simulink model "ModelAgriAuto"  (R2022a)
settings: Solver=FixedStepAuto  StartTime=0.0  StopTime=6240  FixedStep=0.05  MaxStep=0.1  RelTol=1e-3
model workspace (MAT data in the model file):
  PlowHectare = 1.925
values from neighbouring files (symbols this model uses):
  C_rate = 3    [start_function.m]
  Compaction = 0    [start_function.m]
  CyclesIn = CyclesIn+CyclesOut(end)    [start_function.m]
  Degradation = 2    [start_function.m]
  FailRate = 29700000    [start_function.m]
  FieldEff = 0.8    [start_function.m]
  ForceCorrVar = 0.85    [start_function.m]
  Fuel = 3    [start_function.m]
  Mass = 10550    [start_function.m]
  n = n+1    (= 2)    [start_function.m]
  v_field = 5    [start_function.m]
  Weather_crit = 3    [start_function.m]
  WorkingHours = 10    [start_function.m]
undefined symbols (not defined in the file or in its folder): Battery, BatteryNo, Charger, ChargerNo, DField, m, Power, Soil, TractorNo, Year
libraries: simulink x2
(part 3 of 3)

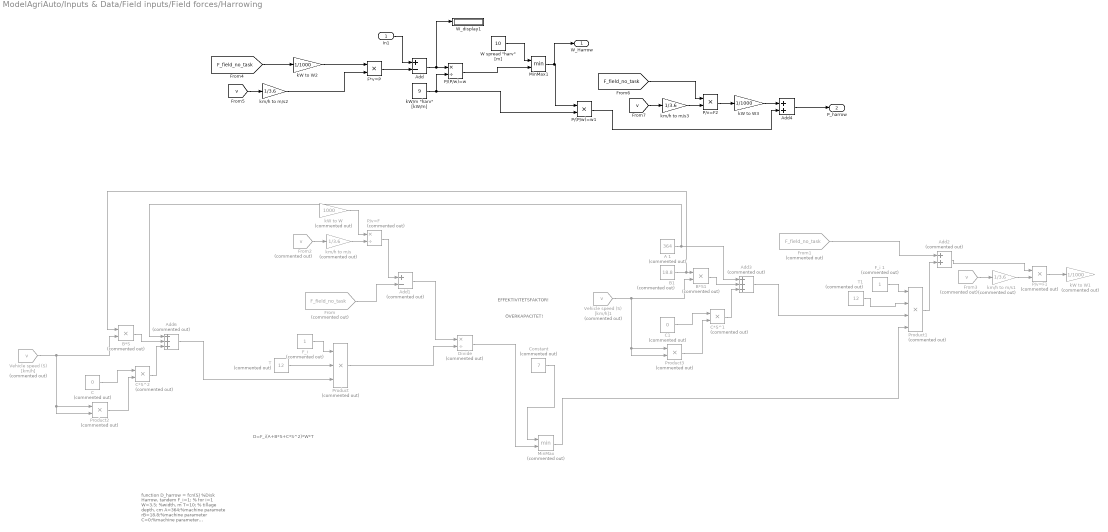
== system ModelAgriAuto/Inputs & Data/Field inputs/Field forces/Harrowing ==
  note: function D_harrow = fcn(S)
      |
      | %Disk Harrow, tandem
      | F_i=1; % for i=1
      | W=3.5; %width, m
      | T=10; % tillage depth, cm
      | A=364;%machine paramete
      | rB=18.8;%machine parameter
      | C=0;%machine parameter
      |
      | D_harrow=F_i*(A+B*S+C*S^2)*W*T;
  note: EFFEKTIVITETSFAKTOR!
  note: ÖVERKAPACITET!
  note: D=F_i(A+B*S+C*S^2)*W*T
  In1 : Inport
  A 1 : Constant  Commented=on  Value=364
  Add : Sum  Inputs=+-
  Add1 : Sum  Commented=on  Inputs=+-
  Add2 : Sum  Commented=on
  Add3 : Sum  Commented=on  Inputs=+++
  Add4 : Sum
  Add6 : Sum  Commented=on  Inputs=+++
  B*S : Product  Commented=on
  B*S1 : Product  Commented=on
  B1 : Constant  Commented=on  Value=18.8
  C : Constant  Commented=on  Value=0
  C*S^1 : Product  Commented=on
  C*S^2 : Product  Commented=on
  C1 : Constant  Commented=on  Value=0
  Constant : Constant  Commented=on  Value=7
  Divide : Product  Commented=on  Inputs=*/
  F*v=P : Product  Inputs=**
  "F_i " : Constant  Commented=on
  F_i 1 : Constant  Commented=on
  From : From  Commented=on  GotoTag=F_field_no_task  TagVisibility=global
  From1 : From  Commented=on  GotoTag=F_field_no_task  TagVisibility=global
  From2 : From  Commented=on  GotoTag=v  TagVisibility=global
  From3 : From  Commented=on  GotoTag=v  TagVisibility=global
  MinMax : MinMax  Commented=on  Inputs=2
  MinMax1 : MinMax  Inputs=2
  P/(P/w)=w : Product  Inputs=*/
  P/(P/w)=w1 : Product  Inputs=**
  P/v=F : Product  Commented=on  Inputs=*/
  P/v=F1 : Product  Commented=on  Inputs=**
  P/v=F2 : Product  Inputs=**
  Product : Product  Commented=on  Inputs=3
  Product1 : Product  Commented=on  Inputs=4
  Product2 : Product  Commented=on
  Product3 : Product  Commented=on
  T : Constant  Commented=on  Value=12
  T1 : Constant  Commented=on  Value=12
  Vehicle speed (S) [km/h] : From  Commented=on  GotoTag=v  TagVisibility=global
  Vehicle speed (S) [km/h]1 : From  Commented=on  GotoTag=v  TagVisibility=global
  "W spread \"harv\" [m]" : Constant  Value=10
  W_display1 : Display
  kW to W : Gain  Commented=on  Gain=1000
  kW to W1 : Gain  Commented=on  Gain=1/1000
  kW to W2 : Gain  Gain=1/1000
  kW to W3 : Gain  Gain=1/1000
  "kW/m \"harv\" [kW/m] " : Constant  Value=9
  km/h to m/s : Gain  Commented=on  Gain=1/3.6
  km/h to m/s1 : Gain  Commented=on  Gain=1/3.6
  km/h to m/s2 : Gain  Gain=1/3.6
  km/h to m/s3 : Gain  Gain=1/3.6
  W_Harrow : Outport  VectorParamsAs1DForOutWhenUnconnected=off
  P_harrow : Outport  Port=2  VectorParamsAs1DForOutWhenUnconnected=off
  wires:
  Product2/1 -> C*S^2/2
  T/1 -> Product/2
  C/1 -> C*S^2/1
  C*S^2/1 -> Add6/3
  From/1 -> Add1/2
  km/h to m/s/1 -> P/v=F/2
  kW to W/1 -> P/v=F/1
  Vehicle speed (S) [km/h]/1 -> Product2/2, Product2/1, B*S/2
  Add1/1 -> Divide/1
  "F_i "/1 -> Product/1
  Product/1 -> Divide/2
  Add6/1 -> Product/3
  B*S/1 -> Add6/2
  From2/1 -> km/h to m/s/1
  B1/1 -> B*S/1, B*S1/1
  A 1/1 -> Add6/1, Add3/1
  Divide/1 -> MinMax/2
  Constant/1 -> MinMax/1
  P/v=F/1 -> Add1/1
  B*S1/1 -> Add3/2
  Product3/1 -> C*S^1/2
  C*S^1/1 -> Add3/3
  F_i 1/1 -> Product1/1
  C1/1 -> C*S^1/1
  Vehicle speed (S) [km/h]1/1 -> Product3/2, Product3/1, B*S1/2
  Add2/1 -> P/v=F1/1
  T1/1 -> Product1/2
  MinMax/1 -> Product1/4
  Add3/1 -> Product1/3
  Product1/1 -> Add2/2
  From1/1 -> Add2/1
  km/h to m/s1/1 -> P/v=F1/2
  From3/1 -> km/h to m/s1/1
  P/v=F1/1 -> kW to W1/1
  F*v=P/1 -> Add/2
  "W spread \"harv\" [m]"/1 -> MinMax1/1
  [F_field_no_task] -> kW to W2/1
  [v] -> km/h to m/s2/1
  P/(P/w)=w/1 -> MinMax1/2
  km/h to m/s2/1 -> F*v=P/2
  kW to W2/1 -> F*v=P/1
  Add/1 -> W_display1/1, P/(P/w)=w/1
  P/(P/w)=w1/1 -> Add4/2
  MinMax1/1 -> W_Harrow/1, P/(P/w)=w1/1
  "kW/m \"harv\" [kW/m] "/1 -> P/(P/w)=w1/2, P/(P/w)=w/2
  [v] -> km/h to m/s3/1
  [F_field_no_task] -> P/v=F2/1
  km/h to m/s3/1 -> P/v=F2/2
  P/v=F2/1 -> kW to W3/1
  kW to W3/1 -> Add4/1
  In1/1 -> Add/1
  Add4/1 -> P_harrow/1

== system ModelAgriAuto/Inputs & Data/Field inputs/Field forces/Motion resistance  ==
  note: %rho =MR/W=1/B_n+0.04+ 0.5*s/sqrtBn
  Add : Sum  Inputs=+++
  B_n : Constant  Value=55
  Constant : Constant  Value=1000
  Constant1 : Constant
  Constant2 : Constant  Value=0.04
  Constant4 : Constant  Value=0.5
  Divide : Product  Inputs=*/
  Divide1 : Product  Inputs=**/
  Divide2 : Product  Inputs=/*
  Product1 : Product
  Product2 : Product
  Sqrt : Sqrt
  g : Constant  Value=9.81
  kN to N : Gain  Gain=1000
  "slippage " : Constant  Value=0.2
  tag scope: MR=global
  wires:
  B_n/1 -> Sqrt/1, Divide/2
  Constant1/1 -> Divide/1
  [m] -> Divide1/1
  g/1 -> Divide1/2
  Divide/1 -> Add/1
  Constant2/1 -> Add/2
  Constant4/1 -> Product1/1
  "slippage "/1 -> Product1/2
  Sqrt/1 -> Divide2/1
  Product1/1 -> Divide2/2
  Divide2/1 -> Add/3
  Add/1 -> Product2/2
  Divide1/1 -> Product2/1
  Product2/1 -> kN to N/1
  Constant/1 -> Divide1/3
  kN to N/1 -> [MR]

== system ModelAgriAuto/Inputs & Data/Field inputs/Field forces/Pest Spreading ==
  note: EMMA och Engström/Lagnelöv 2017
  In2 : Inport
  Add : Sum  Inputs=+-
  Add4 : Sum
  Constant1 : Constant  Commented=on  Value=3.1159
  Constant2 : Constant  Commented=on  Value=2.33
  F*v=P : Product  Inputs=**
  MinMax : MinMax  Inputs=2
  "P spread \"fastgödsel\" [kW]" : Constant  Commented=on  Value=48
  "P spread \"kletgödsel\" [kW]" : Constant  Commented=on  Value=43
  "P spread \"konstgödsel\" [kW]" : Constant  Commented=on  Value=16
  "P spread \"urin\" [kW] " : Constant  Commented=on  Value=28
  P/(P/w)=w : Product  Inputs=*/
  P/(P/w)=w1 : Product  Inputs=**
  P/v=F2 : Product  Inputs=**
  "W spread \"art. fert.\" [m]" : Constant  Value=24
  "W spread \"fastgödsel\" [m]" : Constant  Commented=on  Value=6
  "W spread \"kletgödsel\" [m]1" : Constant  Commented=on  Value=13.8
  "W spread \"konstgödsel\" [m]" : Constant  Commented=on  Value=22
  "W spread \"urin\" [m]" : Constant  Commented=on  Value=12
  W_display1 : Display
  "ha/h \"kletgödsel\" " : Constant  Commented=on  Value=6.9
  "ha/h \"konstgödsel\" " : Constant  Commented=on  Value=11
  kW to W1 : Gain  Gain=1/1000
  kW to W3 : Gain  Gain=1/1000
  kW/m : Constant  Commented=on  Value=0.7273
  "kW/m \"Urin\" [kW/m] " : Constant  Value=2.2917
  km/h to m/s1 : Gain  Gain=1/3.6
  km/h to m/s3 : Gain  Gain=1/3.6
  kw/m : Constant  Commented=on  Value=8
  W_spread : Outport  VectorParamsAs1DForOutWhenUnconnected=off
  P_spread : Outport  Port=2  VectorParamsAs1DForOutWhenUnconnected=off
  wires:
  In2/1 -> Add/1
  [F_field_no_task] -> kW to W1/1
  MinMax/1 -> P/(P/w)=w1/1, W_spread/1
  "W spread \"art. fert.\" [m]"/1 -> MinMax/1
  kW to W1/1 -> F*v=P/1
  [v] -> km/h to m/s1/1
  km/h to m/s1/1 -> F*v=P/2
  F*v=P/1 -> Add/2
  Add/1 -> W_display1/1, P/(P/w)=w/1
  "kW/m \"Urin\" [kW/m] "/1 -> P/(P/w)=w1/2, P/(P/w)=w/2
  P/(P/w)=w/1 -> MinMax/2
  P/v=F2/1 -> kW to W3/1
  kW to W3/1 -> Add4/1
  [F_field_no_task] -> P/v=F2/1
  km/h to m/s3/1 -> P/v=F2/2
  [v] -> km/h to m/s3/1
  P/(P/w)=w1/1 -> Add4/2
  Add4/1 -> P_spread/1

== system ModelAgriAuto/Inputs & Data/Field inputs/Field forces/Plowing ==
  note: Moldboard Plow
  note: W=1; %width, m
      | F_i=1; % for i=1
      | T=20; % tillage depth, cm
      | A=652;%machine paramete
      | B=0;%machine parameter
      | C=5.1;%machine parameter
  note: D=F_i(A+B*S+C*S^2)*W*T
  In1 : Inport
  "A " : Constant  Value=652
  Add1 : Sum  Inputs=+-
  Add2 : Sum
  Add6 : Sum  Inputs=+++
  B : Constant  Value=0
  B*S : Product
  C : Constant  Value=5.1
  C*S^2 : Product
  Constant : Constant  Value=6
  Display : Display
  Divide : Product  Inputs=*/
  MinMax : MinMax  Inputs=2
  P/v=F : Product  Inputs=*/
  Product : Product  Inputs=3
  Product{1..2,4..5} (4 alike) : Product
  T : Constant  Value=20
  W to kW1 : Gain  Gain=1/1000
  W to kW2 : Gain  Gain=1/1000
  kW to W : Gain  Gain=1000
  km/h to m/s : Gain  Gain=1/3.6
  km/h to m/s1 : Gain  Gain=1/3.6
  W_Plow : Outport  VectorParamsAs1DForOutWhenUnconnected=off
  P_plow : Outport  Port=2  VectorParamsAs1DForOutWhenUnconnected=off
  tag scope: P_no_task=global
  wires:
  Product/1 -> Product1/1, Divide/2
  Product2/1 -> C*S^2/2
  B*S/1 -> Add6/2
  C*S^2/1 -> Add6/3
  [F_i] -> Product/1
  [v] -> Product2/2, Product2/1, B*S/2
  km/h to m/s/1 -> P/v=F/2
  T/1 -> Product/2
  "A "/1 -> Add6/1
  kW to W/1 -> P/v=F/1
  B/1 -> B*S/1
  C/1 -> C*S^2/1
  P/v=F/1 -> Add1/1
  [v] -> km/h to m/s/1
  In1/1 -> kW to W/1
  Divide/1 -> MinMax/2
  [F_field_no_task] -> Add1/2
  Add1/1 -> Divide/1
  MinMax/1 -> W_Plow/1, Product1/2
  Constant/1 -> MinMax/1
  Add6/1 -> Product/3
  [F_field_no_task] -> Product5/1, Add2/1
  km/h to m/s1/1 -> Product5/2, Product4/2
  [v] -> km/h to m/s1/1
  Add2/1 -> Product4/1
  Product1/1 -> Add2/2
  W to kW1/1 -> P_plow/1
  W to kW2/1 -> Display/1, [P_no_task]
  Product4/1 -> W to kW1/1
  Product5/1 -> W to kW2/1

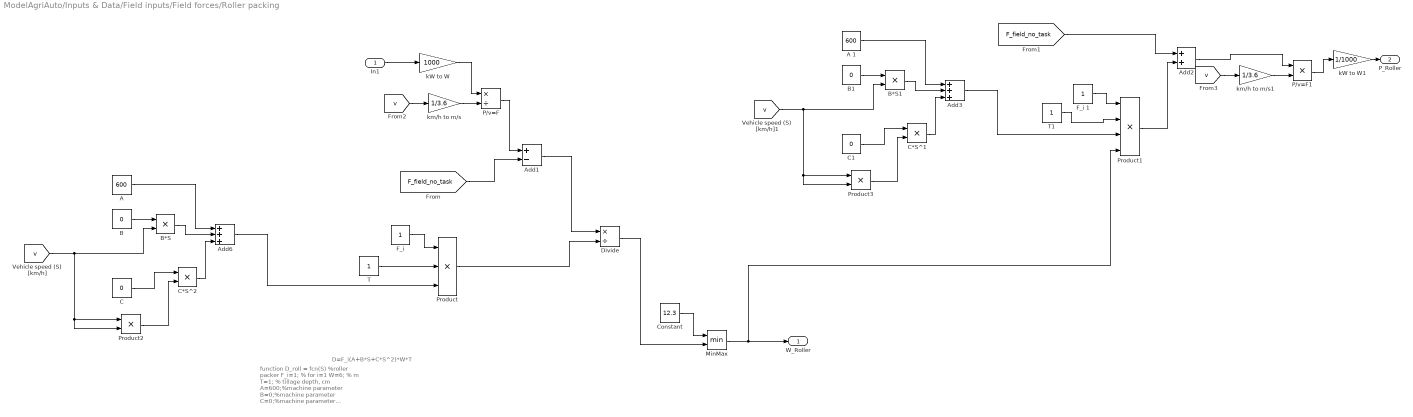
== system ModelAgriAuto/Inputs & Data/Field inputs/Field forces/Roller packing ==
  note: function D_roll = fcn(S)
      |
      | %roller packer
      |
      | F_i=1; % for i=1
      | W=6; % m
      | T=1; % tillage depth, cm
      | A=600;%machine parameter
      | B=0;%machine parameter
      | C=0;%machine parameter
      |
      | D_roll=F_i*(A+B*S+C*S^2)*W*T;
  note: D=F_i(A+B*S+C*S^2)*W*T
  In1 : Inport
  "A " : Constant  Value=600
  A 1 : Constant  Value=600
  Add1 : Sum  Inputs=+-
  Add2 : Sum
  Add3 : Sum  Inputs=+++
  Add6 : Sum  Inputs=+++
  B : Constant  Value=0
  B*S : Product
  B*S1 : Product
  B1 : Constant  Value=0
  C : Constant  Value=0
  C*S^1 : Product
  C*S^2 : Product
  C1 : Constant  Value=0
  Constant : Constant  Value=12.3
  Divide : Product  Inputs=*/
  "F_i " : Constant
  F_i 1 : Constant
  MinMax : MinMax  Inputs=2
  P/v=F : Product  Inputs=*/
  P/v=F1 : Product  Inputs=**
  Product : Product  Inputs=3
  Product1 : Product  Inputs=4
  Product2 : Product
  Product3 : Product
  T : Constant
  T1 : Constant
  kW to W : Gain  Gain=1000
  kW to W1 : Gain  Gain=1/1000
  km/h to m/s : Gain  Gain=1/3.6
  km/h to m/s1 : Gain  Gain=1/3.6
  W_Roller : Outport  VectorParamsAs1DForOutWhenUnconnected=off
  P_Roller : Outport  Port=2  VectorParamsAs1DForOutWhenUnconnected=off
  wires:
  "A "/1 -> Add6/1
  B/1 -> B*S/1
  [v] -> km/h to m/s/1
  B*S/1 -> Add6/2
  Add6/1 -> Product/3
  Product/1 -> Divide/2
  "F_i "/1 -> Product/1
  C/1 -> C*S^2/1
  kW to W/1 -> P/v=F/1
  km/h to m/s/1 -> P/v=F/2
  [F_field_no_task] -> Add1/2
  Add1/1 -> Divide/1
  [v] -> Product2/2, Product2/1, B*S/2
  In1/1 -> kW to W/1
  Product2/1 -> C*S^2/2
  C*S^2/1 -> Add6/3
  T/1 -> Product/2
  Divide/1 -> MinMax/2
  Constant/1 -> MinMax/1
  P/v=F/1 -> Add1/1
  MinMax/1 -> Product1/4, W_Roller/1
  A 1/1 -> Add3/1
  T1/1 -> Product1/2
  C1/1 -> C*S^1/1
  Product3/1 -> C*S^1/2
  Add2/1 -> P/v=F1/1
  kW to W1/1 -> P_Roller/1
  Product1/1 -> Add2/2
  Add3/1 -> Product1/3
  [v] -> Product3/2, Product3/1, B*S1/2
  B*S1/1 -> Add3/2
  [F_field_no_task] -> Add2/1
  B1/1 -> B*S1/1
  F_i 1/1 -> Product1/1
  C*S^1/1 -> Add3/3
  [v] -> km/h to m/s1/1
  km/h to m/s1/1 -> P/v=F1/2
  P/v=F1/1 -> kW to W1/1

== system ModelAgriAuto/Inputs & Data/Field inputs/Field forces/Rolling resistance force calculator ==
  m : Inport
  Rolling resistance calculator : MATLAB Function  TreatAsAtomicUnit=on
  F_rr_field : Outport  VectorParamsAs1DForOutWhenUnconnected=off
  wires:
  m/1 -> Rolling resistance calculator/1(m)
  Rolling resistance calculator/1(F_rr_field) -> F_rr_field/1

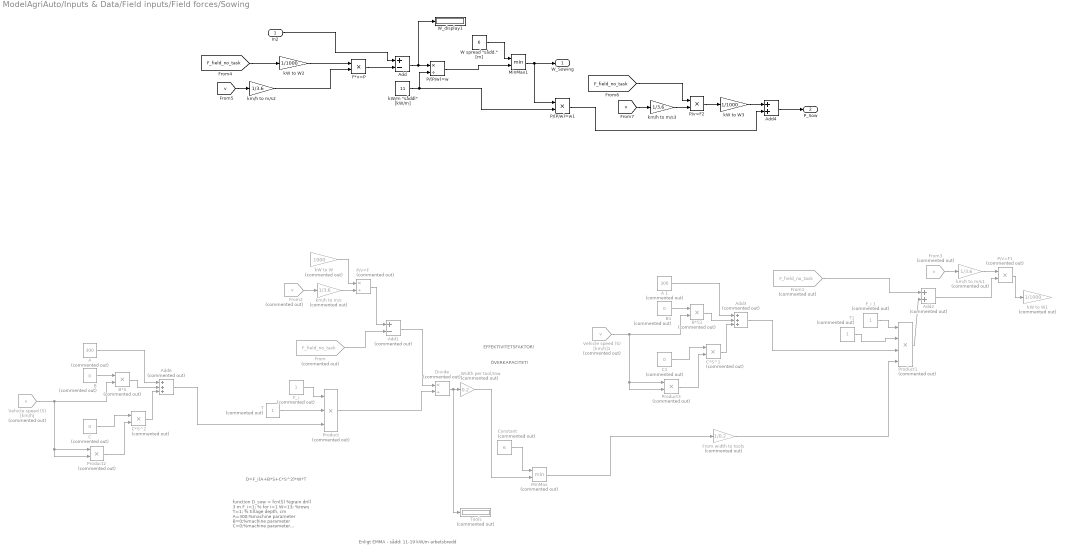
== system ModelAgriAuto/Inputs & Data/Field inputs/Field forces/Sowing ==
  note: Enligt EMMA - sådd: 11-19 kW/m arbetsbredd
  note: function D_sow = fcn(S)
      |
      | %grain drill 3 m
      |
      | F_i=1; % for i=1
      | W=13; %rows
      | T=1; % tillage depth, cm
      | A=300;%machine parameter
      | B=0;%machine parameter
      | C=0;%machine parameter
      |
      | D_sow=F_i*(A+B*S+C*S^2)*W*T;
  note: D=F_i(A+B*S+C*S^2)*W*T
  note: ÖVERKAPACITET!
  note: EFFEKTIVITETSFAKTOR!
  In2 : Inport
  "A " : Constant  Commented=on  Value=300
  A 1 : Constant  Commented=on  Value=300
  Add : Sum  Inputs=+-
  Add1 : Sum  Commented=on  Inputs=+-
  Add2 : Sum  Commented=on
  Add3 : Sum  Commented=on  Inputs=+++
  Add4 : Sum
  Add6 : Sum  Commented=on  Inputs=+++
  B : Constant  Commented=on  Value=0
  B*S : Product  Commented=on
  B*S1 : Product  Commented=on
  B1 : Constant  Commented=on  Value=0
  C : Constant  Commented=on  Value=0
  C*S^1 : Product  Commented=on
  C*S^2 : Product  Commented=on
  C1 : Constant  Commented=on  Value=0
  Constant : Constant  Commented=on  Value=6
  Divide : Product  Commented=on  Inputs=*/
  F*v=P : Product  Inputs=**
  "F_i " : Constant  Commented=on
  F_i 1 : Constant  Commented=on
  From : From  Commented=on  GotoTag=F_field_no_task  TagVisibility=global
  From width to tools : Gain  Commented=on  Gain=1/0.2
  From1 : From  Commented=on  GotoTag=F_field_no_task  TagVisibility=global
  From2 : From  Commented=on  GotoTag=v  TagVisibility=global
  From3 : From  Commented=on  GotoTag=v  TagVisibility=global
  MinMax : MinMax  Commented=on  Inputs=2
  MinMax1 : MinMax  Inputs=2
  P/(P/w)=w : Product  Inputs=*/
  P/(P/w)=w1 : Product  Inputs=**
  P/v=F : Product  Commented=on  Inputs=*/
  P/v=F1 : Product  Commented=on  Inputs=**
  P/v=F2 : Product  Inputs=**
  Product : Product  Commented=on  Inputs=3
  Product1 : Product  Commented=on  Inputs=4
  Product2 : Product  Commented=on
  Product3 : Product  Commented=on
  T : Constant  Commented=on
  T1 : Constant  Commented=on
  Tools : Display  Commented=on
  Vehicle speed (S) [km/h] : From  Commented=on  GotoTag=v  TagVisibility=global
  Vehicle speed (S) [km/h]1 : From  Commented=on  GotoTag=v  TagVisibility=global
  "W spread \"sådd.\" [m]" : Constant  Value=6
  W_display1 : Display
  Width per tool/row : Gain  Commented=on  Gain=0.2
  kW to W : Gain  Commented=on  Gain=1000
  kW to W1 : Gain  Commented=on  Gain=1/1000
  kW to W2 : Gain  Gain=1/1000
  kW to W3 : Gain  Gain=1/1000
  "kW/m \"såddl\" [kW/m] " : Constant  Value=11
  km/h to m/s : Gain  Commented=on  Gain=1/3.6
  km/h to m/s1 : Gain  Commented=on  Gain=1/3.6
  km/h to m/s2 : Gain  Gain=1/3.6
  km/h to m/s3 : Gain  Gain=1/3.6
  W_Sowing : Outport  VectorParamsAs1DForOutWhenUnconnected=off
  P_Sow : Outport  Port=2  VectorParamsAs1DForOutWhenUnconnected=off
  wires:
  "A "/1 -> Add6/1
  B/1 -> B*S/1
  From2/1 -> km/h to m/s/1
  B*S/1 -> Add6/2
  Add6/1 -> Product/3
  Product/1 -> Divide/2
  "F_i "/1 -> Product/1
  Divide/1 -> Tools/1, Width per tool/row/1
  C/1 -> C*S^2/1
  kW to W/1 -> P/v=F/1
  km/h to m/s/1 -> P/v=F/2
  From/1 -> Add1/2
  Add1/1 -> Divide/1
  Vehicle speed (S) [km/h]/1 -> Product2/2, Product2/1, B*S/2
  Product2/1 -> C*S^2/2
  C*S^2/1 -> Add6/3
  T/1 -> Product/2
  Width per tool/row/1 -> MinMax/2
  Constant/1 -> MinMax/1
  P/v=F/1 -> Add1/1
  MinMax/1 -> From width to tools/1
  B1/1 -> B*S1/1
  B*S1/1 -> Add3/2
  C*S^1/1 -> Add3/3
  F_i 1/1 -> Product1/1
  From1/1 -> Add2/1
  Add3/1 -> Product1/3
  Product1/1 -> Add2/2
  Vehicle speed (S) [km/h]1/1 -> Product3/2, Product3/1, B*S1/2
  T1/1 -> Product1/2
  Add2/1 -> P/v=F1/2
  Product3/1 -> C*S^1/2
  C1/1 -> C*S^1/1
  A 1/1 -> Add3/1
  From width to tools/1 -> Product1/4
  km/h to m/s1/1 -> P/v=F1/1
  From3/1 -> km/h to m/s1/1
  P/v=F1/1 -> kW to W1/1
  "W spread \"sådd.\" [m]"/1 -> MinMax1/1
  "kW/m \"såddl\" [kW/m] "/1 -> P/(P/w)=w1/2, P/(P/w)=w/2
  km/h to m/s2/1 -> F*v=P/2
  P/(P/w)=w/1 -> MinMax1/2
  F*v=P/1 -> Add/2
  Add/1 -> W_display1/1, P/(P/w)=w/1
  [F_field_no_task] -> kW to W2/1
  [v] -> km/h to m/s2/1
  kW to W2/1 -> F*v=P/1
  MinMax1/1 -> P/(P/w)=w1/1, W_Sowing/1
  In2/1 -> Add/1
  P/(P/w)=w1/1 -> Add4/2
  kW to W3/1 -> Add4/1
  [v] -> km/h to m/s3/1
  km/h to m/s3/1 -> P/v=F2/2
  [F_field_no_task] -> P/v=F2/1
  Add4/1 -> P_Sow/1
  P/v=F2/1 -> kW to W3/1

== system ModelAgriAuto/Inputs & Data/Field inputs/Fieldwork choice & data/Havre // Oats ==
  note: 15 mars-31 oktober
  note: (Growing period: 1512-4104 h)
  note: Summer period: 2208-2976 h -- Spread
  note: Post-harvest period: 4104-5592 h -- Plow, Cultivate
  note: Spring period: 0-1512 h -- Cultivate, Harrow, Spread, Harrow, Sow, Roller
  note: sladd, harv, kgsprid, harv, så, vält, kgsprid, spruta, skörd, stubb
  note: Oats - Task order
      |
      | 1: Cultivate/ "sladda"
      | 2: Harrow / Harva
      | 3: Fertilizer Spreading/Gödsling
      | 4: Harrow / Harva
      | 5: Sow / Så
      | 6: Roller packing / Vältning
      | ----
      | 7: Herb/pesticide Spreading / Ogräsbekämpning
      | ----
      | 8: Cultivating / Kultivering
      | 9: Plow / Plöja
  Task matrix : Constant  Value="[2 3 2 4 5 7\t0 7 1 0 0 0 0\t0 0 6]"
  Oats : Outport  VectorParamsAs1DForOutWhenUnconnected=off
  wires:
  Task matrix/1 -> Oats/1

== system ModelAgriAuto/Inputs & Data/Field inputs/Fieldwork choice & data/Höstvete // Winter Wheat ==
  note: kgsprid, kgsprid, spruta, skörd, stubb, sladd, vält, kgsprid, harv, harv, så
  "X " : Constant  Value="[0\t0\t0\t0\t0\t7\t3\t7\t\t1\t1\t5\t3\t2\t2\t4\t0]"
  Winter Wheat : Outport  VectorParamsAs1DForOutWhenUnconnected=off
  wires:
  "X "/1 -> Winter Wheat/1

== system ModelAgriAuto/Inputs & Data/Field inputs/Fieldwork choice & data/Korn // Barley ==
  note: sladd, harv, kgsprid, harv, så, vält, kgsprid, spruta, skörd,plog
  "X " : Constant  Value="[2\t3\t2\t4\t5\t7\t0\t7\t\t0\t0\t0\t0\t0\t0\t0\t6]"
  Barley : Outport  VectorParamsAs1DForOutWhenUnconnected=off
  wires:
  "X "/1 -> Barley/1

== system ModelAgriAuto/Inputs & Data/Field inputs/Fieldwork choice & data/Subsystem ==
  In1 : Inport
  Multiport Switch : MultiPortSwitch  Inputs=7  DiagnosticForDefault=None  SaturateOnIntegerOverflow=off  InputSameDT=off
  Multiport Switch1 : MultiPortSwitch  Inputs=7  DiagnosticForDefault=None  SaturateOnIntegerOverflow=off  InputSameDT=off
  P : Outport  VectorParamsAs1DForOutWhenUnconnected=off
  W : Outport  Port=2  VectorParamsAs1DForOutWhenUnconnected=off
  wires:
  [W_plow] -> Multiport Switch1/7
  [W_roll] -> Multiport Switch1/6
  [W_harrow] -> Multiport Switch1/3
  [W_cultivate] -> Multiport Switch1/2
  [W_sow] -> Multiport Switch1/5
  Multiport Switch/1 -> P/1
  [W_spread] -> Multiport Switch1/4
  In1/1 -> Multiport Switch1/1, Multiport Switch/1
  Multiport Switch1/1 -> W/1
  [P_cultivate] -> Multiport Switch/2
  [P_harrow] -> Multiport Switch/3
  [P_sow] -> Multiport Switch/5
  [P_spread] -> Multiport Switch/4
  [P_roller] -> Multiport Switch/6
  [P_plow] -> Multiport Switch/7
  [P_spread_pest] -> Multiport Switch/8
  [W_spread_pest] -> Multiport Switch1/8

== system ModelAgriAuto/Inputs & Data/Field inputs/Fieldwork choice & data/Vårvete // Spring wheat ==
  note: sladd, harv, kgsprid, harv, så, vält, kgsprid, spruta, skörd,plog
  note: sladd, harv, kgsprid, harv, så, vält, kgsprid, spruta, skörd,plog
  "X " : Constant  Value="[2\t3\t2\t4\t5\t7\t0\t7\t\t0\t0\t0\t0\t0\t0\t0\t6]"
  Spring Wheat : Outport  VectorParamsAs1DForOutWhenUnconnected=off
  wires:
  "X "/1 -> Spring Wheat/1

== system ModelAgriAuto/Time & Weather subsyst./Weather & schedule subsystem/Daily soil water content model /Q_d (drainage [mm//day]) ==
  Day to hour 4 : Gain  Gain=1/24
  Display : Display
  Divide : Product  Inputs=*/
  Divide1 : Product  Inputs=**
  Drainage rate exponent : Subsystem
  Math Function2 : Math  Operator=pow  SignedPower=on
  "Q_d " : Outport  VectorParamsAs1DForOutWhenUnconnected=off
  wires:
  [K_FC] -> Divide1/1
  [m_p] -> Divide/1
  Drainage rate exponent/1("Drainage rate exponent ") -> Display/1, Math Function2/2
  Divide/1 -> Math Function2/1
  Math Function2/1 -> Divide1/2
  Divide1/1 -> Day to hour 4/1
  Day to hour 4/1 -> "Q_d "/1
  [FC] -> Divide/2

== system ModelAgriAuto/Time & Weather subsyst./Weather & schedule subsystem/Daily soil water content model /Q_e (Evotranspiration [mm//day])  ==
  note: Från Whitney och SMHI
  Chart : Stateflow chart  TreatAsAtomicUnit=on
  Clock : Clock
  Constant : Constant  Value=0.005
  Constant4 : Constant
  Day to hour 2 : Gain  Gain=1/24
  Demux : Demux  Outputs=8
  Display{,1..4} (5 alike) : Display
  Divide : Product  Inputs=**
  Divide1 : Product  Inputs=*****
  E_p (potential evotranspiration rate) Witney : Subsystem
  Gain : Gain  Gain=1/30
  If dry proceding day : Constant  Value=1.6
  If rainy proceding day : Constant  Value=0.5
  K_d (soil dryness factor) : Subsystem
  K_g : Constant  Value=0.5
  K_l * K_w : Product
  K_s : Sum  Inputs=+-
  K_w : Switch  Criteria=u2 > Threshold  SaturateOnIntegerOverflow=off  InputSameDT=off
  Multiport Switch : MultiPortSwitch  Inputs=8  SaturateOnIntegerOverflow=off  InputSameDT=off
  Scope2 : Scope
  Scope3 : Scope
  Y : Constant  Value=15
  Out1 : Outport  VectorParamsAs1DForOutWhenUnconnected=off
  tag scope: t_n=global
  wires:
  Y/1 -> Divide/2
  Constant/1 -> Divide/1
  Constant4/1 -> K_s/1
  Divide/1 -> K_s/2
  K_s/1 -> Display2/1, Divide1/3
  K_g/1 -> Divide1/2
  K_w/1 -> K_l * K_w/1
  If dry proceding day/1 -> K_w/3
  [Q_p] -> K_w/2
  Chart/1(t_n) -> [t_n], Multiport Switch/1
  Clock/1 -> Chart/1(t)
  Demux/4 -> Multiport Switch/5
  Demux/2 -> Multiport Switch/3
  Demux/5 -> Multiport Switch/6
  Demux/6 -> Multiport Switch/7
  Demux/7 -> Multiport Switch/8
  Demux/3 -> Multiport Switch/4
  Demux/8 -> Multiport Switch/9
  Demux/1 -> Multiport Switch/2
  Multiport Switch/1 -> K_l * K_w/2
  If rainy proceding day/1 -> K_w/1
  K_l * K_w/1 -> Display1/1, Divide1/5
  E_p (potential evotranspiration rate) Witney/1(E_p) -> Display4/1, Scope2/1, Divide1/1
  Divide1/1 -> Gain/1
  Gain/1 -> Day to hour 2/1
  K_d (soil dryness factor)/1(F) -> Display3/1, Scope3/1, Divide1/4
  Day to hour 2/1 -> Out1/1, Display/1
  [K_l] -> Demux/1

== system ModelAgriAuto/Time & Weather subsyst./Weather & schedule subsystem/Daily soil water content model /Q_p (precipitation [mm//day])  ==
  In1 : Inport
  Gain : Gain  Gain=24
  Out1 : Outport  VectorParamsAs1DForOutWhenUnconnected=off
  tag scope: Q_p=global
  wires:
  In1/1 -> Gain/1, Out1/1
  Gain/1 -> [Q_p]

== system ModelAgriAuto/Time & Weather subsyst./Weather & schedule subsystem/Daily soil water content model /Q_r (Runoff [mm//day]) ==
  Add : Sum  Inputs=++-
  Add1 : Sum  Inputs=+-
  Add2 : Sum  Inputs=+-
  Constant : Constant  Value=529
  Constant1 : Constant  Value=2.44
  Constant2 : Constant  Value=2.85
  Constant3 : Constant  Value=615
  Day to hour 3 : Gain  Gain=1/24
  Display{,1..4} (5 alike) : Display
  Divide : Product  Inputs=**
  Divide1 : Product  Inputs=*/
  Divide2 : Product  Inputs=**
  Divide3 : Product  Inputs=**
  "I_m ( Antecendent Soil Moisture index [mm]) " : Subsystem
  Q_r : Outport  VectorParamsAs1DForOutWhenUnconnected=off
  wires:
  [Q_p] -> Add1/1, Divide2/1, Add/1
  Constant/1 -> Add/2
  Constant1/1 -> Divide/1
  "I_m ( Antecendent Soil Moisture index [mm]) "/1(Out1) -> Display/1, Divide3/2, Divide/2
  Divide/1 -> Add/3
  Add/1 -> Display2/1, Divide1/2
  Constant3/1 -> Add2/1
  Constant2/1 -> Divide3/1
  Divide3/1 -> Add2/2
  Add2/1 -> Display1/1, Divide2/2
  Divide2/1 -> Divide1/1
  Divide1/1 -> Display3/1, Add1/2
  Add1/1 -> Display4/1, Day to hour 3/1
  Day to hour 3/1 -> Q_r/1

== system ModelAgriAuto/Time & Weather subsyst./Weather & schedule subsystem/Daily soil water content model /m_p (Moisture content previous day [mm]) ==
  In1 : Inport
  Out1 : Outport  VectorParamsAs1DForOutWhenUnconnected=off
  wires:
  In1/1 -> Out1/1

== system ModelAgriAuto/Time & Weather subsyst./Weather & schedule subsystem/Daily soil water content model /Q_d (drainage [mm//day])/Drainage rate exponent ==
  Add1 : Sum  Inputs=+-
  Add2 : Sum  Inputs=+-
  Divide : Product  Inputs=*/
  Math Function{,1..3} (4 alike) : Math  Operator=log  SignedPower=on
  "Drainage rate exponent " : Outport  VectorParamsAs1DForOutWhenUnconnected=off
  wires:
  [K_SAT] -> Math Function1/1
  [K_FC] -> Math Function/1
  Math Function1/1 -> Add2/1
  Math Function/1 -> Add2/2
  Add2/1 -> Divide/1
  Math Function2/1 -> Add1/1
  Math Function3/1 -> Add1/2
  Add1/1 -> Divide/2
  Divide/1 -> "Drainage rate exponent "/1
  [SAT] -> Math Function2/1
  [FC] -> Math Function3/1

== system ModelAgriAuto/Time & Weather subsyst./Weather & schedule subsystem/Daily soil water content model /Q_e (Evotranspiration [mm//day]) /E_p (potential evotranspiration rate) Witney ==
  Constant : Constant  Value=16
  Constant1 : Constant  Value=10
  Display{,1..4} (5 alike) : Display
  Divide : Product  Inputs=*/
  Math Function : Math  Operator=pow  SignedPower=on
  Product : Product
  Product1 : Product
  T_a (Mean monthly air temperature) : Subsystem
  evaporation rate exponent (beta) : Subsystem
  E_p : Outport  VectorParamsAs1DForOutWhenUnconnected=off
  wires:
  Constant/1 -> Product/1
  Constant1/1 -> Product1/1
  T_a (Mean monthly air temperature)/1(T_a) -> Display3/1, Divide/1
  Divide/1 -> Product1/2
  Product1/1 -> Display4/1, Math Function/1
  [i_h] -> Display/1, evaporation rate exponent (beta)/1(i_h), Divide/2
  Product/1 -> E_p/1
  Math Function/1 -> Display1/1, Product/2
  evaporation rate exponent (beta)/1(beta) -> Display2/1, Math Function/2
  [t_n] -> T_a (Mean monthly air temperature)/1(t_n)

== system ModelAgriAuto/Time & Weather subsyst./Weather & schedule subsystem/Daily soil water content model /Q_e (Evotranspiration [mm//day]) /K_d (soil dryness factor) ==
  Add1 : Sum  Inputs=+-
  Add2 : Sum  Inputs=+-
  Constant2 : Constant  Value=1.25
  Constant3 : Constant
  Constant4 : Constant  Value=0
  Divide2 : Product  Inputs=*/
  Product : Product
  Switch : Switch  Criteria=u2 > Threshold  Threshold=0.8  SaturateOnIntegerOverflow=off  InputSameDT=off
  Switch4 : Switch  Criteria=u2 > Threshold  SaturateOnIntegerOverflow=off  InputSameDT=off
  Transport Delay : TransportDelay  DelayTime=0.1
  F : Outport  VectorParamsAs1DForOutWhenUnconnected=off
  wires:
  Add2/1 -> Divide2/2
  Add1/1 -> Switch4/1, Switch4/2
  [m_a] -> Transport Delay/1
  Constant2/1 -> Product/2
  Divide2/1 -> Product/1, Switch/2
  Product/1 -> Switch/3
  Constant3/1 -> Switch/1
  Switch/1 -> F/1
  Transport Delay/1 -> Add1/1
  [PWP] -> Add1/2
  [SAT] -> Add2/1
  [PWP] -> Add2/2
  Constant4/1 -> Switch4/3
  Switch4/1 -> Divide2/1

== system ModelAgriAuto/Time & Weather subsyst./Weather & schedule subsystem/Daily soil water content model /Q_r (Runoff [mm//day])/I_m ( Antecendent Soil Moisture index [mm])  ==
  Add : Sum  Inputs=+-
  Display1 : Display
  Divide : Product  Inputs=**/
  "Soil bulk density factor " : Constant  Value=100
  Out1 : Outport  VectorParamsAs1DForOutWhenUnconnected=off
  wires:
  "Soil bulk density factor "/1 -> Divide/3
  [m_p] -> Add/1
  Divide/1 -> Add/2, Display1/1
  [d_soil] -> Divide/2
  Add/1 -> Out1/1
  [PWP_i] -> Divide/1

== system ModelAgriAuto/Time & Weather subsyst./Weather & schedule subsystem/Daily soil water content model /Q_e (Evotranspiration [mm//day]) /E_p (potential evotranspiration rate) Witney/T_a (Mean monthly air temperature) ==
  note: Från Whitney och SMHI
  t_n : Inport
  Demux : Demux  Outputs=8
  Multiport Switch : MultiPortSwitch  Inputs=8  SaturateOnIntegerOverflow=off  InputSameDT=off
  T_a : Outport  VectorParamsAs1DForOutWhenUnconnected=off
  wires:
  Demux/8 -> Multiport Switch/9
  Demux/3 -> Multiport Switch/4
  Demux/6 -> Multiport Switch/7
  Demux/4 -> Multiport Switch/5
  Demux/5 -> Multiport Switch/6
  [T_a] -> Demux/1
  Demux/7 -> Multiport Switch/8
  Demux/2 -> Multiport Switch/3
  Demux/1 -> Multiport Switch/2
  t_n/1 -> Multiport Switch/1
  Multiport Switch/1 -> T_a/1

== system ModelAgriAuto/Time & Weather subsyst./Weather & schedule subsystem/Daily soil water content model /Q_e (Evotranspiration [mm//day]) /E_p (potential evotranspiration rate) Witney/evaporation rate exponent (beta) ==
  i_h : Inport
  Add : Sum  Inputs=+-++
  Constant : Constant  Value=0.675
  Constant1 : Constant  Value=17900
  Constant2 : Constant  Value=77.1
  Constant3 : Constant  Value=1e-6
  Constant4 : Constant  Value=492000
  Product : Product  Inputs=4
  Product1 : Product  Inputs=3
  Product2 : Product
  Product3 : Product
  beta : Outport  VectorParamsAs1DForOutWhenUnconnected=off
  wires:
  Constant/1 -> Product/1
  i_h/1 -> Product2/1, Product1/2, Product1/1, Product/2, Product/3, Product/4
  Constant2/1 -> Product1/3
  Constant1/1 -> Product2/2
  Constant3/1 -> Product3/2
  Product/1 -> Add/1
  Product1/1 -> Add/2
  Product2/1 -> Add/3
  Constant4/1 -> Add/4
  Add/1 -> Product3/1
  Product3/1 -> beta/1

== stateflow chart ModelAgriAuto/Time & Weather subsyst./Weather & schedule subsystem/Daily soil water content model /Q_e (Evotranspiration [mm//day]) /Chart ==
  state Month
    state March
      entry: t_n=1;
    state April
      entry: t_n=t_n+1;
    state May
      entry: t_n=t_n+1;
    state June
      entry: t_n=t_n+1;
    state September
      entry: t_n=t_n+1;
    state October
      entry: t_n=t_n+1;
    state July
      entry: t_n=t_n+1;
    state August
      entry: t_n=t_n+1;
    (default) -> March
    March -> April : [t>360]
    May -> June : [t>1824]
    April -> May : [t>1080]
    June -> July : [t>2544]
    August -> September : [t>4008]
    July -> August : [t>3288]
    September -> October : [t>4752]
  (default) -> Month
  data: t input; t_n output

== stateflow chart ModelAgriAuto/States & SoC/Chart ==
  state State
    entry: SoCchange=0;
    state ChargeState
      during:SoCchange=Charger;
      during:State=-1;
    state NoState
      during: SoCchange=0;
      during: State=0;
    state RoadState
      during:SoCchange=-P_road;
      during:State= 1;
    state FieldworkState
      during: SoCchange=-P_fieldwork;
      during:State=2;
    (default) -> NoState
    ChargeState -> NoState : [CCblock<=0 & BESblock<=0]
    NoState -> ChargeState [order 1] : [BESblock>=1 || CCblock>=1]
    FieldworkState -> NoState : [Nblock<=0]
    NoState -> FieldworkState [order 2] : [Nblock>0]
    RoadState -> NoState : [Nroad_1<=0]
    NoState -> RoadState [order 3] : [Nroad_1>0 ]
  (default) -> State
  data: Nblock input; CCblock input; BESblock input; Nroad_1 input; P_fieldwork input; P_road input; Charger input; SoCchange output; State output

== matlab function ModelAgriAuto/Inputs & Data/Field inputs/Field forces/Acceleration force calculator/MATLAB Function ==
  data: a input; F_a_field output
function F_a_field = fcn(a)

m=3200; %kg

F_a_field = a*m;

== matlab function ModelAgriAuto/Inputs & Data/Field inputs/Field forces/Drag force calculator/MATLAB Function ==
  data: v input; F_drag_field output
function F_drag_field = fcn(v)

A=2*2; %assuming 2x2 m frontal area
C_D=0.9; %usual coeff for trucks, assuming same
ro_air=1.225; %at sea level 15 Centigrades

F_drag_field = ro_air*(v./3.6).^2*C_D*A*1/2;

== matlab function ModelAgriAuto/Inputs & Data/Field inputs/Field forces/Gradient force calculator1/MATLAB Function ==
  data: grad input; F_grad_field output
function F_grad_field = fcn(grad)
m=3200 ;%kg
grad=grad*pi/180; % degrees in radians
m_i=0; %vikt redskap
N=(m+m_i)*9.81;


F_grad_field = N*sin(grad);

== stateflow chart ModelAgriAuto/Fieldwork Subsystem/Field Subsystem/Chart ==
  state State
    entry: N= 1; %Field number parameter
    entry: X=1; %Task number parameter
    entry: H_out=0;
    entry: X_max=X_1+X_2+X_3;
    entry: Time=zeros(1,18);
    entry: WorkPrev=0;
    during: Time(1,X)=T;
    state GrowingPeriod1
      during: GateControl=0;
      entry: T_temp=T;
      during: T_1=T-T_temp;
      during:WorkOut=0;
      during:WorkTemp=0;
    state TransitionState1
    state SpringPeriod
      entry:Size=FieldSize(N);
      entry: WorkTemp=0;
      during: WorkOut=WorkSpeed*N_Block;
      during:WorkTemp=WorkIn-WorkPrev;
      during: GateControl=1;
      exit: H_out=H_out+Size;
      exit:WorkPrev=WorkIn;
    state Start
    state SummerPeriod
      entry:Size=FieldSize(N);
      entry: WorkTemp=0;
      during: WorkOut=WorkSpeed*N_Block;
      during:WorkTemp=WorkIn-WorkPrev;
      during: GateControl=1;
      exit: H_out=H_out+Size;
      exit:WorkPrev=WorkIn;
    state Post_HarvestPeriod
      entry:Size=FieldSize(N);
      entry: WorkTemp=0;
      during: WorkOut=WorkSpeed*N_Block;
      during:WorkTemp=WorkIn-WorkPrev;
      during: GateControl=1;
      exit: H_out=H_out+Size;
      exit:WorkPrev=WorkIn;
    state GrowingPeriod2
      during: GateControl=0;
      entry: T_temp=T;
      during: T_2=T-T_temp;
      during:WorkOut=0;
      during:WorkTemp=0;
    state TransitionState2
    state End
      during: GateControl=0;
      entry: T_temp=T;
      during: T_3=T-T_temp;
      during:WorkOut=0;
      during:WorkTemp=0;
    state TransitionState3
    GrowingPeriod1 -> SummerPeriod : [T>=2185]
    TransitionState1 -> GrowingPeriod1 [order 1] : [X>X_1]{N=1;}
    SpringPeriod -> TransitionState1 [order 1] : [WorkTemp>=Size]
    (default) -> Start
    SpringPeriod -> TransitionState1 [order 2] : [X_val==0]
    TransitionState1 -> (junction 65) [order 2] : [X<=X_1]{N=N+1;}
    Start -> SpringPeriod : [Workability>0]{TimeSpring=T;}
    (junction 65) -> SpringPeriod [order 1] : [N<=N_max]
    (junction 65) -> (junction 62) [order 2] : [N>N_max]{X=X+1;}
    (junction 62) -> SpringPeriod : {N=1;}
    SummerPeriod -> TransitionState2 [order 1] : [WorkTemp>=Size]
    SummerPeriod -> TransitionState2 [order 2] : [X_val==0]
    (junction 79) -> SummerPeriod [order 2] : [N<=N_max]
    (junction 81) -> SummerPeriod : {N=1;}
    TransitionState2 -> (junction 79) [order 2] : [X<=(X_1+X_2)]{N=N+1;}
    (junction 79) -> (junction 81) [order 1] : [N>N_max]{X=X+1;}
    Post_HarvestPeriod -> TransitionState3 [order 1] : [X_val==0]
    GrowingPeriod2 -> Post_HarvestPeriod : [T>=4057]{TimeFall=T;}
    TransitionState2 -> GrowingPeriod2 [order 1] : [X>(X_1+X_2)]
        | {N=1;}
    Post_HarvestPeriod -> TransitionState3 [order 2] : [WorkTemp>=Size]
    (junction 95) -> Post_HarvestPeriod [order 2] : [N<=N_max]
    (junction 94) -> Post_HarvestPeriod : {N=1;}
    TransitionState3 -> End [order 2] : [X>X_max]
        | {N=1;}
    TransitionState3 -> (junction 95) [order 1] : [X<=X_max]{N=N+1;}
    (junction 95) -> (junction 94) [order 1] : [N>N_max]{X=X+1;}
  (default) -> State
  data: FieldSize input; X output; GateControl output; N output; H_out output; T input; X_1 input; X_2 input; X_3 input; X_max local; N_max input; N_Block input; Size output; T_1 output; T_2 output; T_3 output; T_temp local; X_val input; Time output size=1, 18 [1..17]; WorkSpeed input; WorkOut output; WorkIn input; Workability input; WorkPrev local; WorkTemp output; TimeSpring output; TimeFall output

== matlab function ModelAgriAuto/Inputs & Data/Field inputs/Field forces/Rolling resistance force calculator/Rolling resistance calculator ==
  data: m input; F_rr_field output
function F_rr_field = fcn(m)
m;
C_rr_field=0.1; %clay soil, careful estimate
m_i=0; %vikt redskap
N=(m+m_i)*9.81;


F_rr_field = C_rr_field*N;

== matlab function ModelAgriAuto/Transport Subsystem/Road forces/Drag force road ==
  data: v input; F_drag_road output
function F_drag_road = fcn(v)

A=2*2; %assuming 2x2 m frontal area
C_D=0.9; %usual coeff for trucks, assuming same
ro_air=1.225; %at sea level 15 Centigrades

F_drag_road = ro_air*(v./3.6).^2*C_D*A*1/2;
